simulink model "scalarControl_Induction_motordrive"  (R2020a)
settings: Solver=ode45  StartTime=0  StopTime=1  MaxStep=Ts  RelTol=1e-3  AbsTol=1e-3  EnableMultiTasking=on
undefined symbols (not defined in the file or in its folder): psis_ref, Ts
libraries: simulink x1
settings Model: Creator=mhinkkan  LastModifiedBy=Dinesh Chandresh
settings SolverCC: AutoScaleAbsTol=off
settings DataIOCC: SaveFormat=Array  SignalLoggingSaveFormat=ModelDataLogs  SaveOutput=off  SignalLogging=off  DSMLogging=off  SaveTime=off  ReturnWorkspaceOutputs=off
settings OptimizationCC: BlockReduction=off  BooleanDataType=off  DefaultParameterBehavior=Inlined  OptimizeBlockIOStorage=off  BufferReuse=off  ExpressionFolding=off  ExpressionDepthLimit=2147483647  LocalBlockOutputs=off  InitFltsAndDblsToZero=on  LifeSpan=inf
settings DebuggingCC: SaveWithParameterizedLinksMsg=none  UnderspecifiedInitializationDetection=Classic  MergeDetectMultiDrivingBlocksExec=none  SignalResolutionControl=TryResolveAllWithWarning  MultiTaskDSMMsg=warning  MultiTaskCondExecSysMsg=none  FcnCallInpInsideContextMsg=warning  StateNameClashWarn=warning  SFUnexpectedBacktrackingDiag=warning  SFNoUnconditionalDefaultTransitionDiag=warning  SFExecutionAtInitializationDiag=none  ArithmeticOperatorsInVariantConditions=warning
settings HardwareCC: ProdBitPerPointer=32  ProdBitPerSizeT=32  ProdBitPerPtrDiffT=32  ProdLargestAtomicFloat=None  ProdIntDivRoundTo=Undefined  ProdEndianess=Unspecified  ProdWordSize=32  ProdHWDeviceType=32-bit Generic  TargetUnknown=on
settings ModelReferenceCC: PropagateSignalLabelsOutOfModel=off
settings SFSimCC: SimUseLocalCustomCode=off  CustomCodeUndefinedFunction=UseInterfaceOnly
settings RTWCC: RTWUseLocalCustomCode=off
settings CodeAppCC: StateflowObjectComments=on
settings GRTTargetCC: TargetFcnLib=ansi_tfl_tmw.mat  TargetLangStandard=C89/C90 (ANSI)  CombineOutputUpdateFcns=off  GRTInterface=on
settings ConfigComp: CovMetricSettings=dw  CovHtmlReporting=on  CovSaveCumulativeToWorkspaceVar=on  CovSaveSingleToWorkspaceVar=on  CovExternalEMLEnable=off

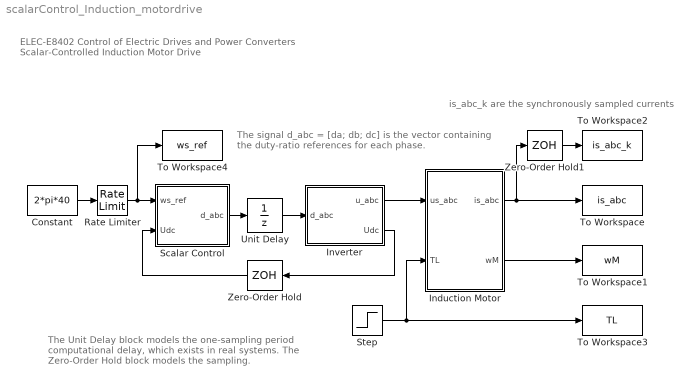
== system scalarControl_Induction_motordrive ==
  note: is_abc_k are the synchronously sampled currents
  note: The signal d_abc = [da; db; dc] is the vector
      | containing the duty-ratio references for each phase.
  note: ELEC-E8402 Control of Electric Drives and Power Converters
      |
      | Scalar-Controlled Induction Motor Drive
  note: The Unit Delay block models the one-sampling period
      | computational delay, which exists in real systems.
      | The Zero-Order Hold block models the sampling.
  Constant : Constant  Value=2*pi*40  SampleTime=Ts
  Induction Motor : Subsystem  mask{Rs=3.7, RR=2.1, Lsigma=21e-3, LM=0.224, p=2, J=0.016}
      mask prompts: Rs "Stator resistance Rs (ohm)"; RR "Rotor resistance RR (ohm)"; Lsigma "Leakage inductance Lsigma (H)"; LM "Magnetizing inductance LM (H)"; p "Number of pole pairs p"; J "Total inertia J (kgm^2)"
      mask help: Inverse-Gamma model
  Inverter : Subsystem  mask{Ts=Ts, Udc=540}
      mask prompts: Ts "Sampling period Ts (s)"; Udc "DC-link voltage Udc (V)"
      mask help: The switching period is 2*Ts and the switching frequency is 1/(2*Ts).
  Rate Limiter : RateLimiter  RisingSlewLimit=2*pi*100  FallingSlewLimit=-2*pi*100  SampleTimeMode=inherited
  Scalar Control : Subsystem
  Step : Step  Time=.6  After=14.6298  SampleTime=0
  To Workspace : ToWorkspace  VariableName=is_abc  SaveFormat=Timeseries  SampleTime=-1
  To Workspace1 : ToWorkspace  VariableName=wM  SaveFormat=Timeseries  SampleTime=-1
  To Workspace2 : ToWorkspace  VariableName=is_abc_k  SaveFormat=Timeseries  SampleTime=-1
  To Workspace3 : ToWorkspace  VariableName=TL  SaveFormat=Timeseries  SampleTime=-1
  To Workspace4 : ToWorkspace  VariableName=ws_ref  SaveFormat=Timeseries  SampleTime=-1
  Unit Delay : UnitDelay  SampleTime=Ts  HasFrameUpgradeWarning=on
  Zero-Order Hold : ZeroOrderHold  SampleTime=Ts
  Zero-Order Hold1 : ZeroOrderHold  SampleTime=Ts
  wires:
  Step/1 -> Induction Motor/2(TL), To Workspace3/1
  Inverter/1(u_abc) -> Induction Motor/1(us_abc)
  Induction Motor/1(is_abc) -> Zero-Order Hold1/1, To Workspace/1
  Induction Motor/2(wM) -> To Workspace1/1
  Unit Delay/1 -> Inverter/1(d_abc)
  Zero-Order Hold/1 -> Scalar Control/2(Udc)
  Scalar Control/1(d_abc) -> Unit Delay/1
  Constant/1 -> Rate Limiter/1
  Rate Limiter/1 -> To Workspace4/1, Scalar Control/1(ws_ref)
  Inverter/2(Udc) -> Zero-Order Hold/1
  Zero-Order Hold1/1 -> To Workspace2/1

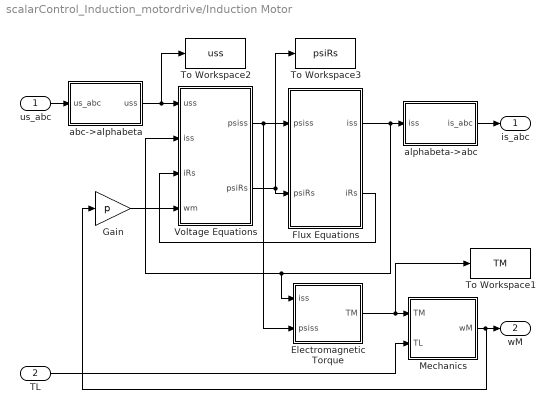
== system scalarControl_Induction_motordrive/Induction Motor ==
  us_abc : Inport
  TL : Inport  Port=2
  Electromagnetic Torque : Subsystem
  Flux Equations : Subsystem
  Gain : Gain  Gain=p  SaturateOnIntegerOverflow=on  OutDataTypeStr=Inherit: Same as input  ParamDataTypeStr=Inherit: Same as input
  Mechanics : Subsystem
  To Workspace1 : ToWorkspace  VariableName=TM  SaveFormat=Timeseries  SampleTime=-1
  To Workspace2 : ToWorkspace  VariableName=uss  SaveFormat=Timeseries  SampleTime=-1
  To Workspace3 : ToWorkspace  VariableName=psiRs  SaveFormat=Timeseries  SampleTime=-1
  Voltage Equations : Subsystem
  abc->alphabeta : Subsystem
  alphabeta->abc : Subsystem
  is_abc : Outport
  wM : Outport  Port=2
  wires:
  TL/1 -> Mechanics/2(TL)
  Mechanics/1(wM) -> wM/1, Gain/1
  Flux Equations/1(iss) -> Voltage Equations/2(iss), Electromagnetic Torque/1(iss), alphabeta->abc/1(iss)
  us_abc/1 -> abc->alphabeta/1(us_abc)
  Voltage Equations/2(psiRs) -> To Workspace3/1, Flux Equations/2(psiRs)
  Voltage Equations/1(psiss) -> Electromagnetic Torque/2(psiss), Flux Equations/1(psiss)
  Flux Equations/2(iRs) -> Voltage Equations/3(iRs)
  Electromagnetic Torque/1(TM) -> To Workspace1/1, Mechanics/1(TM)
  abc->alphabeta/1(uss) -> To Workspace2/1, Voltage Equations/1(uss)
  alphabeta->abc/1(is_abc) -> is_abc/1
  Gain/1 -> Voltage Equations/4(wm)

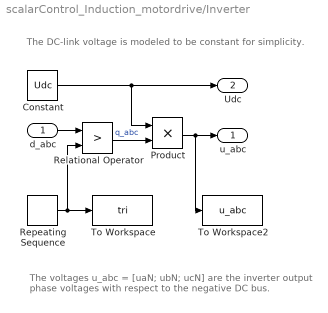
== system scalarControl_Induction_motordrive/Inverter ==
  note: The voltages u_abc = [uaN; ubN; ucN] are the inverter
      | output phase voltages with respect to the negative DC bus.
  note: The DC-link voltage is modeled to be constant for simplicity.
  d_abc : Inport
  Constant : Constant  Value=Udc  SampleTime=0
  Product : Product
  Relational Operator : RelationalOperator  Operator=>  OutDataTypeStr=boolean  RndMeth=Nearest
  Repeating Sequence : simulink/Sources/Repeating Sequence  rep_seq_t=[0 1 2]*Ts  rep_seq_y=[1 0 1]
  To Workspace : ToWorkspace  VariableName=tri  SaveFormat=Timeseries  SampleTime=-1
  To Workspace2 : ToWorkspace  VariableName=u_abc  SaveFormat=Timeseries  SampleTime=-1
  u_abc : Outport
  Udc : Outport  Port=2
  wires:
  Repeating Sequence/1 -> Relational Operator/2, To Workspace/1
  d_abc/1 -> Relational Operator/1
  Relational Operator/1 -> Product/2  "q_abc"
  Constant/1 -> Product/1, Udc/1
  Product/1 -> u_abc/1, To Workspace2/1

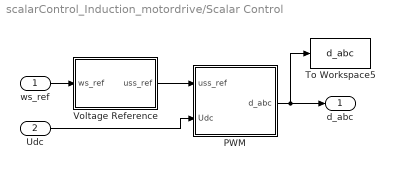
== system scalarControl_Induction_motordrive/Scalar Control ==
  ws_ref : Inport
  Udc : Inport  Port=2
  PWM : Subsystem
  To Workspace5 : ToWorkspace  VariableName=d_abc  SaveFormat=Timeseries  SampleTime=-1
  Voltage Reference : Subsystem
  d_abc : Outport
  wires:
  ws_ref/1 -> Voltage Reference/1(ws_ref)
  Voltage Reference/1(uss_ref) -> PWM/1(uss_ref)
  Udc/1 -> PWM/2(Udc)
  PWM/1(d_abc) -> To Workspace5/1, d_abc/1

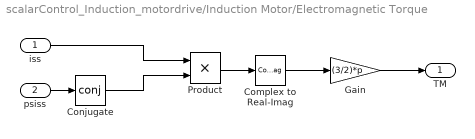
== system scalarControl_Induction_motordrive/Induction Motor/Electromagnetic Torque ==
  iss : Inport
  psiss : Inport  Port=2
  Complex to Real-Imag : ComplexToRealImag  Output=Imag
  Conjugate : Math  Operator=conj  SignedPower=on  RndMeth=Zero  SaturateOnIntegerOverflow=on
  Gain : Gain  Gain=(3/2)*p
  Product : Product
  TM : Outport
  wires:
  psiss/1 -> Conjugate/1
  Conjugate/1 -> Product/2
  iss/1 -> Product/1
  Gain/1 -> TM/1
  Product/1 -> Complex to Real-Imag/1
  Complex to Real-Imag/1 -> Gain/1

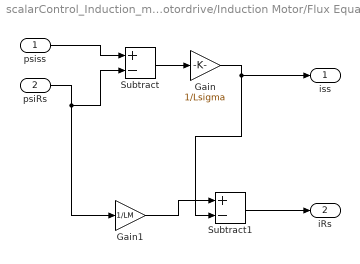
== system scalarControl_Induction_motordrive/Induction Motor/Flux Equations ==
  psiss : Inport
  psiRs : Inport  Port=2
  Gain : Gain  Gain=1/Lsigma
  Gain1 : Gain  Gain=1/LM
  Subtract : Sum  Inputs=+-
  Subtract1 : Sum  Inputs=+-
  iss : Outport
  iRs : Outport  Port=2
  wires:
  psiss/1 -> Subtract/1
  psiRs/1 -> Gain1/1, Subtract/2
  Subtract/1 -> Gain/1
  Gain/1 -> Subtract1/2, iss/1
  Gain1/1 -> Subtract1/1
  Subtract1/1 -> iRs/1

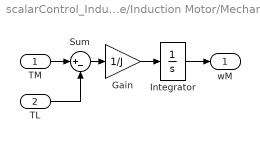
== system scalarControl_Induction_motordrive/Induction Motor/Mechanics ==
  TM : Inport
  TL : Inport  Port=2
  Gain : Gain  Gain=1/J  SaturateOnIntegerOverflow=on  OutDataTypeStr=Inherit: Same as input  ParamDataTypeStr=Inherit: Same as input
  Integrator : Integrator
  Sum : Sum  Inputs=|+-  InputSameDT=on  SaturateOnIntegerOverflow=on  OutDataTypeStr=Inherit: Same as first input
  wM : Outport
  wires:
  TL/1 -> Sum/2
  Sum/1 -> Gain/1
  Gain/1 -> Integrator/1
  Integrator/1 -> wM/1
  TM/1 -> Sum/1

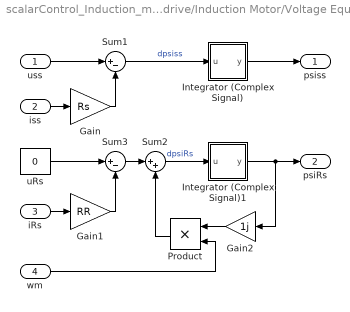
== system scalarControl_Induction_motordrive/Induction Motor/Voltage Equations ==
  uss : Inport
  iss : Inport  Port=2
  iRs : Inport  Port=3
  wm : Inport  Port=4
  Gain : Gain  Gain=Rs
  Gain1 : Gain  Gain=RR
  Gain2 : Gain  Gain=1j
  Integrator (Complex Signal) : Subsystem
      mask Display: disp('1/s');
  Integrator (Complex Signal)1 : Subsystem
      mask Display: disp('1/s');
  Product : Product  RndMeth=Zero
  Sum1 : Sum  Inputs=|+-
  Sum2 : Sum  Inputs=|++
  Sum3 : Sum  Inputs=|+-
  uRs : Constant  Value=0  SampleTime=0
  psiss : Outport
  psiRs : Outport  Port=2
  wires:
  uss/1 -> Sum1/1
  iss/1 -> Gain/1
  Sum1/1 -> Integrator (Complex Signal)/1(u)  "dpsiss"
  Gain/1 -> Sum1/2
  Integrator (Complex Signal)/1(y) -> psiss/1
  uRs/1 -> Sum3/1
  iRs/1 -> Gain1/1
  Gain1/1 -> Sum3/2
  Sum3/1 -> Sum2/1
  Sum2/1 -> Integrator (Complex Signal)1/1(u)  "dpsiRs"
  Product/1 -> Sum2/2
  Integrator (Complex Signal)1/1(y) -> psiRs/1, Gain2/1
  Gain2/1 -> Product/1
  wm/1 -> Product/2

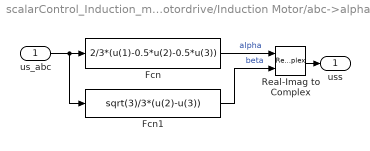
== system scalarControl_Induction_motordrive/Induction Motor/abc->alphabeta ==
  us_abc : Inport
  Fcn : Fcn  Expr=2/3*(u(1)-0.5*u(2)-0.5*u(3))
  Fcn1 : Fcn  Expr=sqrt(3)/3*(u(2)-u(3))
  Real-Imag to Complex : RealImagToComplex
  uss : Outport
  wires:
  us_abc/1 -> Fcn1/1, Fcn/1
  Fcn/1 -> Real-Imag to Complex/1  "alpha"
  Fcn1/1 -> Real-Imag to Complex/2  "beta"
  Real-Imag to Complex/1 -> uss/1

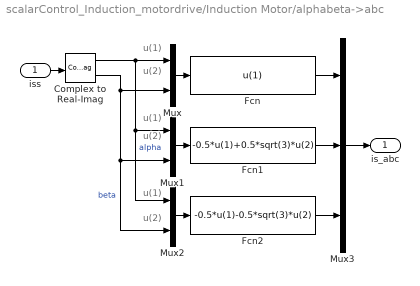
== system scalarControl_Induction_motordrive/Induction Motor/alphabeta->abc ==
  note: u(1)
  note: u(2)
  note: u(1)
  note: u(2)
  note: u(1)
  note: u(2)
  iss : Inport
  Complex to Real-Imag : ComplexToRealImag
  Fcn : Fcn  Expr=u(1)
  Fcn1 : Fcn  Expr=-0.5*u(1)+0.5*sqrt(3)*u(2)
  Fcn2 : Fcn  Expr=-0.5*u(1)-0.5*sqrt(3)*u(2)
  Mux : Mux  Inputs=2
  Mux1 : Mux  Inputs=2
  Mux2 : Mux  Inputs=2
  Mux3 : Mux  Inputs=3
  is_abc : Outport
  wires:
  Mux/1 -> Fcn/1
  Complex to Real-Imag/1 -> Mux/1, Mux1/1, Mux2/1  "alpha"
  Complex to Real-Imag/2 -> Mux/2, Mux1/2, Mux2/2  "beta"
  Mux1/1 -> Fcn1/1
  Mux2/1 -> Fcn2/1
  iss/1 -> Complex to Real-Imag/1
  Fcn/1 -> Mux3/1
  Fcn1/1 -> Mux3/2
  Fcn2/1 -> Mux3/3
  Mux3/1 -> is_abc/1

== system scalarControl_Induction_motordrive/Scalar Control/PWM ==
  note: The signal uss_ref_lim is (the estimate of) the realized
      | voltage space vector. If the modulator does not
      | saturate, uss_ref_lim = uss_ref.
  uss_ref : Inport
  Udc : Inport  Port=2
  MATLAB Function : MATLAB Function  TreatAsAtomicUnit=on
  To Workspace : ToWorkspace  VariableName=uss_ref_lim  SaveFormat=Timeseries  SampleTime=-1
  d_abc : Outport
  wires:
  uss_ref/1 -> MATLAB Function/1(uss_ref)
  Udc/1 -> MATLAB Function/2(Udc)
  MATLAB Function/1(d_abc) -> d_abc/1
  MATLAB Function/2(uss_ref_lim) -> To Workspace/1

== system scalarControl_Induction_motordrive/Scalar Control/Voltage Reference ==
  ws_ref : Inport
  MATLAB Function : MATLAB Function  TreatAsAtomicUnit=on
  Unit Delay : UnitDelay  SampleTime=-1  HasFrameUpgradeWarning=on
  uss_ref : Outport
  wires:
  Unit Delay/1 -> MATLAB Function/2(thetas)
  ws_ref/1 -> MATLAB Function/1(ws_ref)
  MATLAB Function/1(uss_ref) -> uss_ref/1
  MATLAB Function/2(thetas_new) -> Unit Delay/1

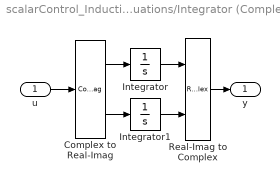
== system scalarControl_Induction_motordrive/Induction Motor/Voltage Equations/Integrator (Complex Signal) ==
  u : Inport
  Complex to Real-Imag : ComplexToRealImag
  Integrator : Integrator
  Integrator1 : Integrator
  Real-Imag to Complex : RealImagToComplex
  y : Outport
  wires:
  Complex to Real-Imag/1 -> Integrator/1
  Complex to Real-Imag/2 -> Integrator1/1
  Integrator/1 -> Real-Imag to Complex/1
  Integrator1/1 -> Real-Imag to Complex/2
  Real-Imag to Complex/1 -> y/1
  u/1 -> Complex to Real-Imag/1

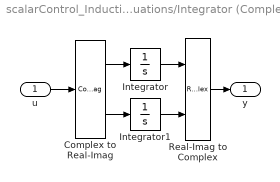
== system scalarControl_Induction_motordrive/Induction Motor/Voltage Equations/Integrator (Complex Signal)1 ==
  u : Inport
  Complex to Real-Imag : ComplexToRealImag
  Integrator : Integrator
  Integrator1 : Integrator
  Real-Imag to Complex : RealImagToComplex
  y : Outport
  wires:
  Complex to Real-Imag/1 -> Integrator/1
  Complex to Real-Imag/2 -> Integrator1/1
  Integrator/1 -> Real-Imag to Complex/1
  Integrator1/1 -> Real-Imag to Complex/2
  Real-Imag to Complex/1 -> y/1
  u/1 -> Complex to Real-Imag/1

== matlab function scalarControl_Induction_motordrive/Scalar Control/PWM/MATLAB Function ==
  data: uss_ref input; Udc input; d_abc output; uss_ref_lim output
function [d_abc,uss_ref_lim] = pwm(uss_ref,Udc)
%#codegen

% Components of the voltage space vector
ualpha_ref = real(uss_ref);
ubeta_ref  = imag(uss_ref);

% Phase-voltage references
ua_ref = ualpha_ref;
ub_ref = .5*(-ualpha_ref + sqrt(3)*ubeta_ref);
uc_ref = .5*(-ualpha_ref - sqrt(3)*ubeta_ref);

% Vector of phase-voltage references
u_abc_ref = [ua_ref; ub_ref; uc_ref];

% Symmetrization of the references by adding the zero-sequence voltage
u0 = .5*(max(u_abc_ref) + min(u_abc_ref));
u_abc_ref = u_abc_ref - u0;

% Clamping of the reference voltages such that no phase error is caused. 
% If all phase voltage reference are realizable (below Udc/2), m = 1 holds.
m = max([2*u_abc_ref/Udc; 1]);
u_abc_ref = u_abc_ref/m;

% Duty cycles, which can be directly used for triangle comparison, 
% if the triangle wave varies between 0...1
d_abc = .5 + u_abc_ref/Udc;

% Realized voltage vector is calculated from the clamped duty ratios.
% If the PWM does not saturate, uss_ref_lim = uss_ref holds. The realized
% voltage vector is needed, e.g., for the current-controller antiwindup.
uss_ref_lim = 2/3*(d_abc(1) + d_abc(2)*exp(1j*2*pi/3) + d_abc(3)*exp(1j*4*pi/3))*Udc;

== matlab function scalarControl_Induction_motordrive/Scalar Control/Voltage Reference/MATLAB Function ==
  data: uss_ref output size=1; ws_ref input size=1; thetas input size=1; psis_ref parameter size=1; Ts parameter size=1; thetas_new output
function [uss_ref,thetas_new]  = scalar(ws_ref,thetas,psis_ref,Ts)
%#codegen

% Voltage vector
% Note: 1j is the imaginary unit in the MATLAB software
 uss_ref =ws_ref*psis_ref*exp(1j*thetas); 	% Complete this 

% Update (integrate) the voltage angle
thetas_new = thetas + Ts*ws_ref;

% Extra information about MATLAB functions: 
% The inputs, ouputs, and parameters of MATLAB functions can be
% defined using "Ports and Data Manager", which can be opened by
% clicking the "Edit Data" button in the toolstrip above. For example, Ts
% and psis_ref are defined to be parameters, which means that their value
% is read from the workspace. In this assignment, you do not need to change
% these settings.
